simulink model "lanelet2_map_provider"  (R2021b)
settings: Solver=FixedStepAuto  StartTime=0.0  StopTime=10.0  RelTol=1e-3
settings Model: Creator=takum  LastModifiedBy=takum
settings OptimizationCC: EnhancedBackFolding=on  PassReuseOutputArgsAs=Individual arguments  ZeroExternalMemoryAtStartup=off  ZeroInternalMemoryAtStartup=off  MaxStackSize=64  OptimizeBlockOrder=speed  DifferentSizesBufferReuse=on  OptimizationCustomize=off  EfficientTunableParamExpr=on
settings DebuggingCC: ParameterTunabilityLossMsg=error
settings SFSimCC: MATLABDynamicMemAlloc=off
settings RTWCC: Description=Embedded Coder  SystemTargetFile=ert.tlc  HardwareBoard=Robot Operating System 2 (ROS 2)  TemplateMakefile=ert_default_tmf  Toolchain=Colcon Tools  TargetLang=C++
settings CodeAppCC: ForceParamTrailComments=on  IgnoreCustomStorageClasses=off  OperatorAnnotations=on  SimulinkDataObjDesc=on  SFDataObjDesc=on  InsertBlockDesc=on
settings ERTTargetCC: CodeInterfacePackaging=C++ class  RootIOFormat=Structure reference

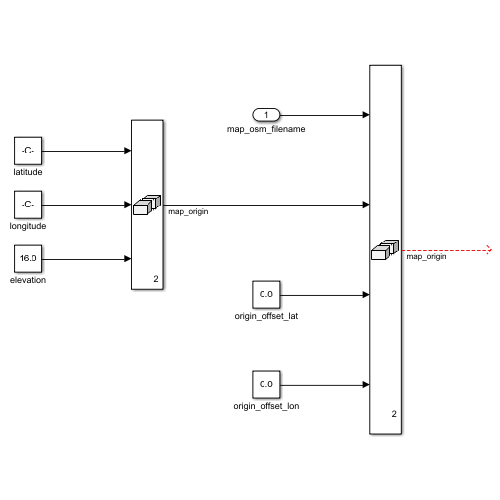
[thumbnail: Simulink's stored preview of the top-level diagram]
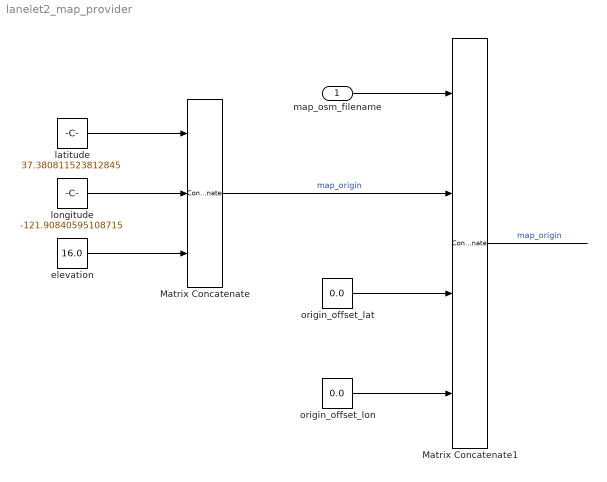
== system lanelet2_map_provider ==
  map_osm_filename : Inport  OutDataTypeStr=string
  Matrix Concatenate : Concatenate  NumInputs=3  Mode=Multidimensional array  ConcatenateDimension=2
  Matrix Concatenate1 : Concatenate  NumInputs=4  Mode=Multidimensional array  ConcatenateDimension=2
  elevation : Constant  Value=16.0
  latitude : Constant  Value=37.380811523812845
  longitude : Constant  Value=-121.90840595108715
  origin_offset_lat : Constant  Value=0.0
  origin_offset_lon : Constant  Value=0.0
  wires:
  latitude/1 -> Matrix Concatenate/1
  longitude/1 -> Matrix Concatenate/2
  elevation/1 -> Matrix Concatenate/3
  Matrix Concatenate/1 -> Matrix Concatenate1/2  "map_origin"
  origin_offset_lat/1 -> Matrix Concatenate1/3
  origin_offset_lon/1 -> Matrix Concatenate1/4
  map_osm_filename/1 -> Matrix Concatenate1/1
  Matrix Concatenate1/1 -> ?  "map_origin"
